simulink model "saildrone"  (R2022a)
settings: Solver=FixedStepAuto  StartTime=0.0  StopTime=10.0  RelTol=1e-3  EnableMultiTasking=on
undefined symbols (not defined in the file): alt, dev, lat, lon, Main, pwm_output0, remaining, voltage_v
libraries: px4Sensorslib x5, px4uORBlib x5, simulink x1, px4lib x1
settings Model: ExtModeTrigDuration=10  Creator=kavin  LastModifiedBy=kavin
settings SolverCC: PositivePriorityOrder=on
settings OptimizationCC: EnhancedBackFolding=on  PassReuseOutputArgsAs=Individual arguments  ZeroExternalMemoryAtStartup=off  ZeroInternalMemoryAtStartup=off  MaxStackSize=64  OptimizeBlockOrder=speed  DifferentSizesBufferReuse=on  OptimizationCustomize=off  EfficientTunableParamExpr=on
settings DebuggingCC: ParameterTunabilityLossMsg=error
settings HardwareCC: ProdBitPerPointer=32  ProdBitPerSizeT=32  ProdBitPerPtrDiffT=32  ProdLargestAtomicInteger=Long  ProdLargestAtomicFloat=Double  ProdWordSize=32  ProdLongLongMode=on  ProdHWDeviceType=ARM Compatible->ARM Cortex
settings SFSimCC: MATLABDynamicMemAlloc=off  SimTargetLang=C++
settings RTWCC: SystemTargetFile=ert.tlc  HardwareBoard=PX4 Pixhawk 4  TLCOptions="-aInlineSetEventsForThisBaseRateFcn=TLC_FALSE -aSuppressMultiTaskScheduler=TLC_FALSE  -aRateBasedStepFcn=0"  TemplateMakefile=ert_default_tmf  Toolchain=GNU Tools for PX4 Autopilots  TargetLang=C++
settings CodeAppCC: ForceParamTrailComments=on  IgnoreCustomStorageClasses=off  OperatorAnnotations=on  SimulinkDataObjDesc=on  SFDataObjDesc=on  InsertBlockDesc=on
settings ERTTargetCC: ExtModeTransport=3  ExtModeStaticAlloc=on  ExtModeStaticAllocSize=1024  ExtModeMexFile=ext_xcp  ExtModeIntrfLevel=Level2 - Open

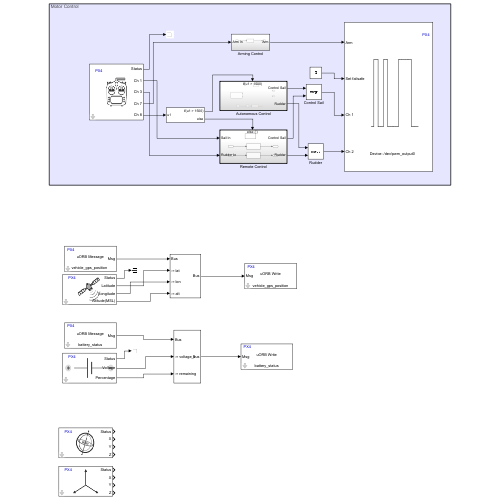
[thumbnail: Simulink's stored preview of the top-level diagram]
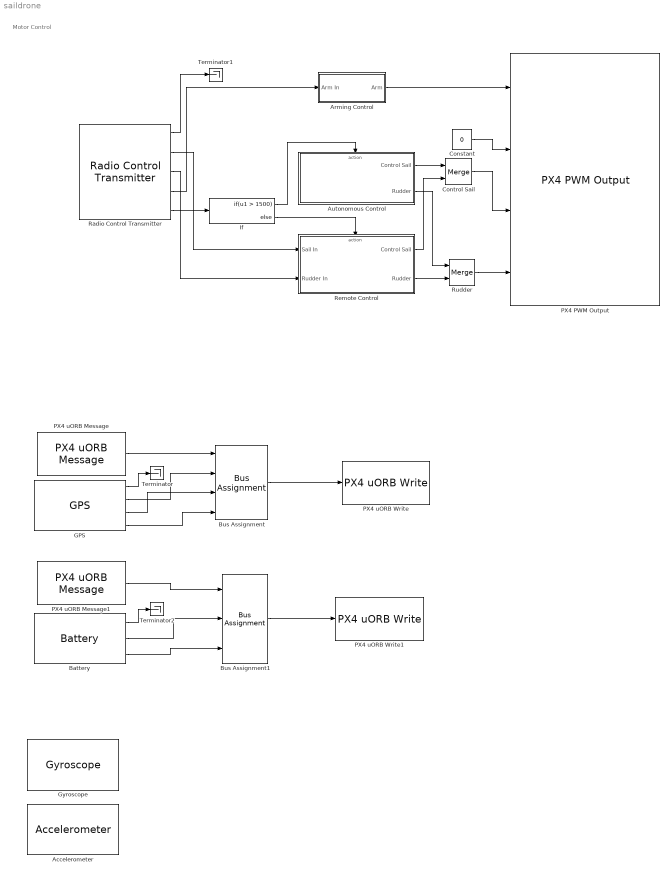
== system saildrone ==
  note: Motor Control
  Accelerometer : px4Sensorslib/Accelerometer  uorbTimeStamp=off  BlockingMode=off  BlockTimeout=1e-3  sampleTime=1/250
      settings: SourceProductBaseCode=PX4AUTOPILOTS
  Arming Control : Subsystem
  Autonomous Control : Subsystem  TreatAsAtomicUnit=on
  Battery : px4Sensorslib/Battery  voltage=on  current=off  remaining=on  warning=off  timestamp=off  sampleTime=1/250  BlockingMode=off  BlockTimeout=1e-3
      settings: SourceProductBaseCode=PX4AUTOPILOTS
  Bus Assignment : BusAssignment  AssignedSignals=lat,lon,alt
  Bus Assignment1 : BusAssignment  AssignedSignals=voltage_v,remaining
  Constant : Constant  Value=0  OutDataTypeStr=boolean
  Control Sail : Merge
  GPS : px4Sensorslib/GPS  lat=on  lon=on  alt=on  velocity=off  course=off  gpsfix=off  numsat=off  timestamp_utc=off  BlockingMode=off  BlockTimeout=1e-3  dop=off  vel_ned=off  alt_ellipsoid=off  jamm_ind=off  timestamp=off  sampleTime=1/250
      settings: SourceProductBaseCode=PX4AUTOPILOTS
  Gyroscope : px4Sensorslib/Gyroscope  uorbTimeStamp=off  BlockingMode=off  BlockTimeout=1e-3  sampleTime=1/250
      settings: SourceProductBaseCode=PX4AUTOPILOTS
  If : If  IfExpression=u1 > 1500
  PX4 PWM Output : px4lib/PX4 PWM Output  pwmDevice=Main (/dev/pwm_output0)  pwmChannel1_=on  pwmChannel2_=on  pwmChannel3_=off  pwmChannel4_=off  pwmChannel5_=off  pwmChannel6_=off  pwmChannel7_=off  pwmChannel8_=off  forceTerminateFailsafe=off  outputErrorStatus=off
      settings: SourceProductBaseCode=PX4AUTOPILOTS
  PX4 uORB Message : px4uORBlib/PX4 uORB Message  uORBTopic=vehicle_gps_position  SampleTime=inf  selectInstance=vehicle_gps_position
      settings: SourceProductBaseCode=PX4AUTOPILOTS
  PX4 uORB Message1 : px4uORBlib/PX4 uORB Message  uORBTopic=battery_status  SampleTime=inf  selectInstance=battery_status
      settings: SourceProductBaseCode=PX4AUTOPILOTS
  PX4 uORB Write : px4uORBlib/PX4 uORB Write  uORBTopic=vehicle_gps_position  selectInstance=vehicle_gps_position  MessageQueueLen=1
      settings: SourceProductBaseCode=PX4AUTOPILOTS
  PX4 uORB Write1 : px4uORBlib/PX4 uORB Write  uORBTopic=battery_status  selectInstance=battery_status  MessageQueueLen=1
      settings: SourceProductBaseCode=PX4AUTOPILOTS
  Radio Control Transmitter : px4Sensorslib/Radio Control Transmitter  channel1=on  channel2=off  channel3=on  channel4=off  channel5=off  channel6=off  channel7=on  channel8=on  channel_count=off  rssi=off  rc_input_source=off  timestamp_last_signal=off  time_stamp=off  sampleTime=1/250  BlockingMode=off  BlockTimeout=5
      settings: SourceProductBaseCode=PX4AUTOPILOTS
  Remote Control : Subsystem  TreatAsAtomicUnit=on
  Rudder : Merge
  Terminator : Terminator
  Terminator1 : Terminator
  Terminator2 : Terminator
  wires:
  If/1 -> Autonomous Control/Action
  If/2 -> Remote Control/Action
  Remote Control/1(Control Sail) -> Control Sail/2
  Remote Control/2(Rudder) -> Rudder/2
  Control Sail/1 -> PX4 PWM Output/3
  Constant/1 -> PX4 PWM Output/2
  Autonomous Control/1(Control Sail) -> Control Sail/1
  Autonomous Control/2(Rudder) -> Rudder/1
  Radio Control Transmitter/5 -> If/1
  Radio Control Transmitter/4 -> Arming Control/1(Arm In)
  Radio Control Transmitter/3 -> Remote Control/2(Rudder In)
  Radio Control Transmitter/2 -> Remote Control/1(Sail In)
  Radio Control Transmitter/1 -> Terminator1/1
  Arming Control/1(Arm) -> PX4 PWM Output/1
  Rudder/1 -> PX4 PWM Output/4
  PX4 uORB Message/1 -> Bus Assignment/1
  GPS/2 -> Bus Assignment/2
  GPS/3 -> Bus Assignment/3
  GPS/4 -> Bus Assignment/4
  Bus Assignment/1 -> PX4 uORB Write/1
  GPS/1 -> Terminator/1
  PX4 uORB Message1/1 -> Bus Assignment1/1
  Bus Assignment1/1 -> PX4 uORB Write1/1
  Battery/2 -> Bus Assignment1/2
  Battery/3 -> Bus Assignment1/3
  Battery/1 -> Terminator2/1

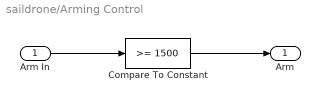
== system saildrone/Arming Control ==
  Arm In : Inport
  Compare To Constant : simulink/Logic and Bit Operations/Compare To Constant  relop=>=  const=1500  OutDataTypeStr=boolean
  Arm : Outport
  wires:
  Arm In/1 -> Compare To Constant/1
  Compare To Constant/1 -> Arm/1

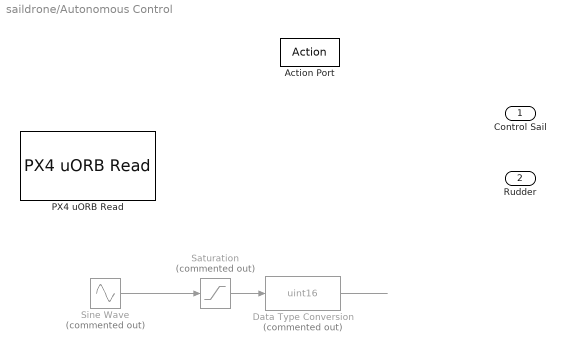
== system saildrone/Autonomous Control ==
  Action Port : ActionPort  ActionPortLabel=if(u1 > 1500)
  Data Type Conversion : DataTypeConversion  Commented=on  OutDataTypeStr=uint16  SaturateOnIntegerOverflow=off  RndMeth=Floor
  PX4 uORB Read : px4uORBlib/PX4 uORB Read  uORBTopic=sensor_accel  selectInstance=sensor_accel  SampleTime=0.001  BlockingMode=off  BlockTimeout=1e-3
      settings: SourceProductBaseCode=PX4AUTOPILOTS
  Saturation : Saturate  Commented=on  UpperLimit=2000  LowerLimit=1000
  Sine Wave : Sin  Commented=on  Amplitude=400  Bias=1500  Frequency=3  SampleTime=0.004
  Control Sail : Outport
  Rudder : Outport  Port=2
  wires:
  Sine Wave/1 -> Saturation/1
  Saturation/1 -> Data Type Conversion/1
  Data Type Conversion/1 -> ?

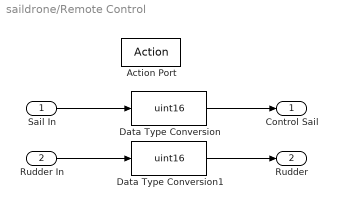
== system saildrone/Remote Control ==
  Sail In : Inport
  Rudder In : Inport  Port=2
  Action Port : ActionPort  ActionPortLabel=else
  Data Type Conversion : DataTypeConversion  OutDataTypeStr=uint16  SaturateOnIntegerOverflow=off  RndMeth=Floor
  Data Type Conversion1 : DataTypeConversion  OutDataTypeStr=uint16  SaturateOnIntegerOverflow=off  RndMeth=Floor
  Control Sail : Outport
  Rudder : Outport  Port=2
  wires:
  Sail In/1 -> Data Type Conversion/1
  Rudder In/1 -> Data Type Conversion1/1
  Data Type Conversion/1 -> Control Sail/1
  Data Type Conversion1/1 -> Rudder/1
